simulink model "PIDonTF"  (R2024b)
settings: Solver=VariableStepAuto  StartTime=0.0  StopTime=1  RelTol=1e-3
values from neighbouring files (symbols this model uses):
  gains = computePIDGains(4, 0.15, 0.1, Ps, "PID")    [reducedPlant.m]
  km = (k_drv*k_t)/((R_eq*B_eq_user) + (k_t*k_e))    [reducedPlant.m]
  N = gbox.N    [reducedPlant.m]
  Tm = (R_eq*J_eq)/((R_eq*B_eq_user) + (k_t*k_e))    [reducedPlant.m]
libraries: simulink_extras x3, slpidlib x1
settings Model: Creator=Nihal  LastModifiedBy=Nihal

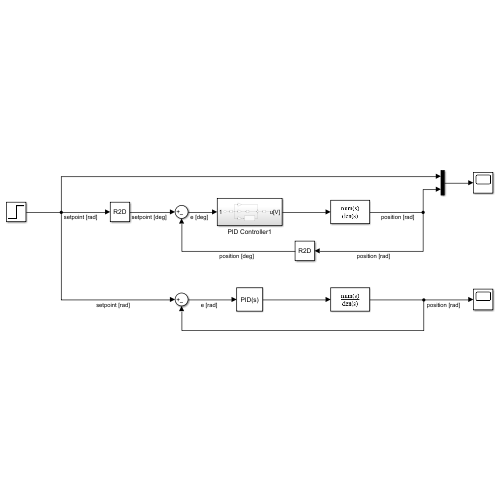
[thumbnail: Simulink's stored preview of the top-level diagram]
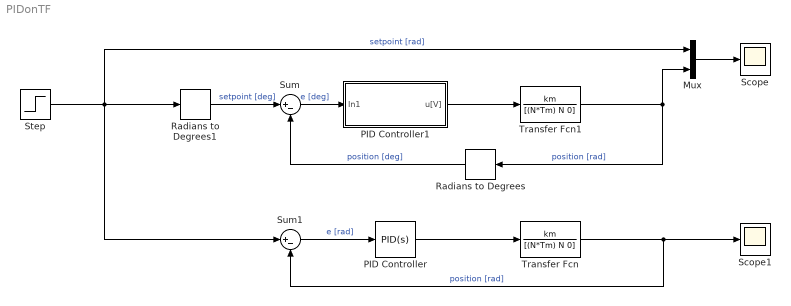
== system PIDonTF ==
  Mux : Mux  Inputs=2
  PID Controller : slpidlib/PID Controller  Controller=PID  Form=Parallel  TimeDomain=Continuous-time  UseExternalTs=off  SampleTime=-1  IntegratorMethod=Forward Euler  FilterMethod=Forward Euler  ControllerParametersSource=internal  P=gains.Kp  I=gains.Ki  UseKiTs=off  D=1.5  UseExternalDerivativeSource=off  N=1/gains.Tl  UseFilter=on  TunerSelectOption=Transfer Function Based (PID Tuner App)  InitialConditionSource=internal  InitialConditionForIntegrator=0  InitialConditionForFilter=0  DifferentiatorICPrevScaledInput=0  ExternalReset=none  TrackingMode=off  Kt=1  LimitOutput=off  SatLimitsSource=internal  UpperSaturationLimit=inf  LowerSaturationLimit=-inf  LinearizeAsGain=on  AntiWindupMode=none  Kb=1  LimitIntegrator=off  UpperIntegratorSaturationLimit=inf  LowerIntegratorSaturationLimit=-inf  POutMin=[]  POutMax=[]  IOutMin=[]  IOutMax=[]  DOutMin=[]  DOutMax=[]  NOutMin=[]  NOutMax=[]  SumOutMin=[]  SumOutMax=[]  SaturationOutMin=[]  SaturationOutMax=[]  PParamMin=[]  PParamMax=[]  IParamMin=[]  IParamMax=[]  DParamMin=[]  DParamMax=[]  NParamMin=[]  NParamMax=[]  KbParamMin=[]  KbParamMax=[]  KtParamMin=[]  KtParamMax=[]  KbOutMin=[]  KbOutMax=[]  KtOutMin=[]  KtOutMax=[]  IntegratorOutMin=[]  IntegratorOutMax=[]  FilterOutMin=[]  FilterOutMax=[]  SumI1OutMin=[]  SumI1OutMax=[]  SumI2OutMin=[]  SumI2OutMax=[]  SumI3OutMin=[]  SumI3OutMax=[]  SumI4OutMin=[]  SumI4OutMax=[]  SumDOutMin=[]  SumDOutMax=[]  DifferentiatorOutMin=[]  DifferentiatorOutMax=[]  FilterDiffOutCoefMin=[]  FilterDiffOutCoefMax=[]  ReciprocalOutMin=[]  ReciprocalOutMax=[]  SumDenOutMin=[]  SumDenOutMax=[]  SumNumOutMin=[]  SumNumOutMax=[]  DivideOutMin=[]  DivideOutMax=[]  UdiffTsProdOutMin=[]  UdiffTsProdOutMax=[]  NTsProdOutMin=[]  NTsProdOutMax=[]  UintegralTsProdOutMin=[]  UintegralTsProdOutMax=[]  UngainTsProdOutMin=[]  UngainTsProdOutMax=[]  ClampingZeroOutDataTypeStr=Inherit: Inherit via back propagation  ClampingZeroOutMin=[]  ClampingZeroOutMax=[]  FilterDenConstantOutDataTypeStr=Inherit: Inherit via back propagation  FilterDenConstantOutMin=[]  FilterDenConstantOutMax=[]  PCopyOutDataTypeStr=Inherit: Inherit via back propagation  PCopyOutMin=[]  PCopyOutMax=[]  NCopyOutDataTypeStr=Inherit: Inherit via back propagation  NCopyOutMin=[]  NCopyOutMax=[]  IntegratorContinuousStateAttributes=''  IntegratorStateMustResolveToSignalObject=off  IntegratorRTWStateStorageClass=Auto  FilterContinuousStateAttributes=''  FilterStateMustResolveToSignalObject=off  FilterRTWStateStorageClass=Auto  ParallelPVariant=InternalParameters  IdealPVariant=Disabled  IVariant=InternalParameters  DVariant=InternalParameters  IntegratorVariant=Continuous  SatVariant=Disabled  AWVariant=Passthrough  PCopyVariant=Disabled  TRVariant=Disabled  FdbkBlocksVariant=Forward  IdealPFdbkVariant=Disabled  SatFdbkVariant=Disabled  DerivativeFilterVariant=ContFilter  NVariant=InternalParameters  NCopyVariant=Disabled  FilterICVariant=InternalICsFilter  IntegratorICVariant=InternalICs  ExternalResetVariant=Disabled  TRSumVariant=Passthrough  SumFdbkVariant=Disabled  SumVariant=Sum_PID  TsampFilterVariant=InternalTs  TsampNgainVariant=Passthrough  TsampIntegralVariant=Disabled_SignalSpec  ExternalSaturationOutDataTypeStr=Inherit: Same as second input  DerivativeSourceVariant=ErrorSignal  PreIntVariant=InternalPreInt
  PID Controller1 : Subsystem
  Radians to Degrees : simulink_extras/Transformations/Radians to Degrees
  Radians to Degrees1 : simulink_extras/Transformations/Radians to Degrees
  Scope : Scope
  Scope1 : Scope
  Step : Step  Time=0  SampleTime=0
  Sum : Sum  Inputs=|+-
  Sum1 : Sum  Inputs=|+-
  Transfer Fcn : TransferFcn  Numerator=km  Denominator=[(N*Tm) N 0]
  Transfer Fcn1 : TransferFcn  Numerator=km  Denominator=[(N*Tm) N 0]
  wires:
  Step/1 -> Radians to Degrees1/1, Sum1/1, Mux/1  "setpoint [rad]"
  Sum/1 -> PID Controller1/1(In1)  "e [deg]"
  PID Controller1/1(u[V]) -> Transfer Fcn1/1
  Mux/1 -> Scope/1
  Transfer Fcn1/1 -> Radians to Degrees/1, Mux/2  "position [rad]"
  Radians to Degrees/1 -> Sum/2  "position [deg]"
  Transfer Fcn/1 -> Sum1/2, Scope1/1  "position [rad]"
  Sum1/1 -> PID Controller/1  "e [rad]"
  PID Controller/1 -> Transfer Fcn/1
  Radians to Degrees1/1 -> Sum/1  "setpoint [deg]"

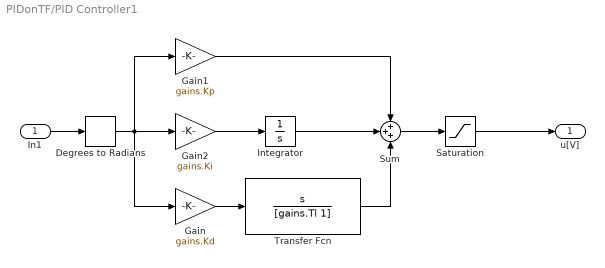
== system PIDonTF/PID Controller1 ==
  In1 : Inport
  Degrees to Radians : simulink_extras/Transformations/Degrees to Radians
  Gain : Gain  Gain=gains.Kd
  Gain1 : Gain  Gain=gains.Kp
  Gain2 : Gain  Gain=gains.Ki
  Integrator : Integrator
  Saturation : Saturate  UpperLimit=12  LowerLimit=-12
  Sum : Sum  Inputs=+++
  Transfer Fcn : TransferFcn  Numerator=[1 0]  Denominator=[gains.Tl 1]
  u[V] : Outport
  wires:
  In1/1 -> Degrees to Radians/1
  Sum/1 -> Saturation/1
  Saturation/1 -> u[V]/1
  Degrees to Radians/1 -> Gain/1, Gain1/1, Gain2/1
  Gain/1 -> Transfer Fcn/1
  Gain2/1 -> Integrator/1
  Transfer Fcn/1 -> Sum/3
  Integrator/1 -> Sum/2
  Gain1/1 -> Sum/1
